simulink model "J544"  (R2015b)
settings: Solver=VariableStepAuto  StartTime=-10  StopTime=10.0  RelTol=1e-3
libraries: simulink x1
settings Model: Creator=Pouya  LastModifiedBy=Pouya

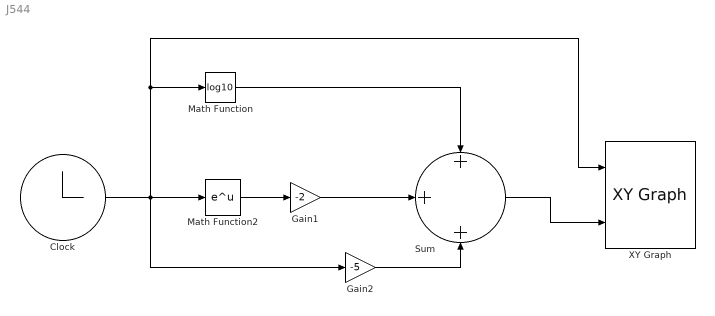
== system J544 ==
  Clock : Clock
  Gain1 : Gain  Gain=-2
  Gain2 : Gain  Gain=-5
  Math Function : Math  Operator=log10  SaturateOnIntegerOverflow=on
  Math Function2 : Math  SaturateOnIntegerOverflow=on
  Sum : Sum  Inputs=+++
  XY Graph : simulink/Sinks/XY Graph  xmin=-10  xmax=10  ymin=-100  ymax=100  st=-1
  wires:
  Clock/1 -> Gain2/1, Math Function/1, XY Graph/1, Math Function2/1
  Math Function2/1 -> Gain1/1
  Math Function/1 -> Sum/1
  Gain1/1 -> Sum/2
  Gain2/1 -> Sum/3
  Sum/1 -> XY Graph/2
